simulink model "sk_R3GDL_2017"  (Simulink 9.1)
settings: Solver=ode45  StartTime=0.0  StopTime=20  MaxStep=1e-3  RelTol=1e-3  EnableMultiTasking=on
values from neighbouring files (symbols this model uses):
  A11 = 0.5    [Estimacion_Parametros_Ideal.m]    (also in Estimacion_Parametros_Real.m = 3; graficas.m)
  A12 = .5    (= 0.5)    [Estimacion_Parametros_Ideal.m]    (also in Estimacion_Parametros_Real.m = 3; graficas.m)
  F11 = 5    [Estimacion_Parametros_Ideal.m]    (also in Estimacion_Parametros_Real.m; graficas.m)
  F12 = 3    [Estimacion_Parametros_Ideal.m]    (also in Estimacion_Parametros_Real.m = 15; graficas.m)
  Ph11 = 0.5    [Estimacion_Parametros_Ideal.m]    (also in Estimacion_Parametros_Real.m = 0; graficas.m)
  Ph12 = 0    [Estimacion_Parametros_Ideal.m]    (also in Estimacion_Parametros_Real.m; graficas.m)
  Tm = 0.001    [Estimacion_Parametros_Ideal.m]    (also in Estimacion_Parametros_Real.m; graficas.m)
settings Model: Creator=mortega  LastModifiedBy=rafap  ExtModeTrigMode=oneshot  ExtModeArmWhenConnect=off
settings DataIOCC: SignalLoggingSaveFormat=ModelDataLogs
settings OptimizationCC: BlockReduction=off  BooleanDataType=off  ExpressionDepthLimit=2147483647  InitFltsAndDblsToZero=on
settings DebuggingCC: SaveWithParameterizedLinksMsg=none  SignalResolutionControl=TryResolveAllWithWarning  MultiTaskDSMMsg=warning  MultiTaskCondExecSysMsg=none  FcnCallInpInsideContextMsg=warning  StateNameClashWarn=warning
settings HardwareCC: TargetUnknown=on
settings GRTTargetCC: TargetFcnLib=ansi_tfl_tmw.mat

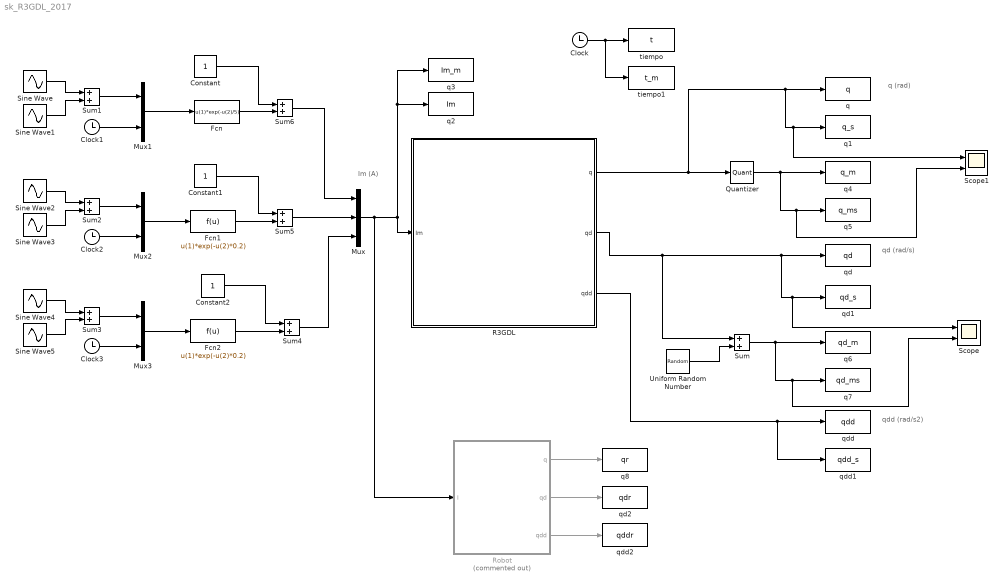
== system sk_R3GDL_2017 ==
  note: Im (A)
  note: q (rad)
  note: qd (rad/s)
  note: qdd (rad/s2)
  Clock{,1..3} (4 alike) : Clock
  Constant : Constant
  Constant1 : Constant
  Constant2 : Constant
  Fcn : Fcn  Expr=u(1)*exp(-u(2)/5)
  Fcn1 : Fcn  Expr=u(1)*exp(-u(2)*0.2)
  Fcn2 : Fcn  Expr=u(1)*exp(-u(2)*0.2)
  Mux : Mux  Inputs=3
  Mux1 : Mux  Inputs=2
  Mux2 : Mux  Inputs=2
  Mux3 : Mux  Inputs=2
  Quantizer : Quantizer  QuantizationInterval=(2*pi)/1024
  R3GDL : Subsystem  mask(Control y Programación de Robots (4 GIERM)){NGrupo=13, q1_ini=0, q2_ini=0, q3_ini=0, Bl_q1=off, Bl_q2=off, Bl_q3=off, AccionamientoDirecto=on}
      mask prompts: NGrupo "Nº de GRUPO"; q1_ini "q1 inicial  (rad)"; q2_ini "q2 inicial (rad)"; q3_ini "q3_inicial (rad)"; Bl_q1 "Bloqueo q1"; Bl_q2 "Bloqueo q2"; Bl_q3 "Bloqueo q3"; AccionamientoDirecto "Accionamiento directo"
      mask help: Robot de 3 grados de libertad RRR
      mask Display:
      | image(imread('R3GDL_RRR.JPG'));
      | port_label('output', 1, 'q');
      | port_label('output', 2, 'qd');
      | port_label('output', 3, 'qdd');
      | port_label('input', 1, 'Im')
  Robot : Subsystem  Commented=on
  Scope : Scope  NumInputPorts=2
  Scope1 : Scope  NumInputPorts=2
  Sine Wave : Sin  Amplitude=A11  Frequency=F11  Phase=Ph11  SampleTime=0
  Sine Wave1 : Sin  Amplitude=A12  Frequency=F12  Phase=Ph12  SampleTime=0
  Sine Wave2 : Sin  Amplitude=A11  Frequency=F11  Phase=Ph11  SampleTime=0
  Sine Wave3 : Sin  Amplitude=A12  Frequency=F12  Phase=Ph12  SampleTime=0
  Sine Wave4 : Sin  Amplitude=A11  Frequency=F11  Phase=Ph11  SampleTime=0
  Sine Wave5 : Sin  Amplitude=A12  Frequency=F12  Phase=Ph12  SampleTime=0
  Sum{,1..6} (7 alike) : Sum
  Uniform Random Number : UniformRandomNumber  Minimum=-0.005  Maximum=0.005  SampleTime=Tm
  q : ToWorkspace  VariableName=q  SampleTime=-1
  q1 : ToWorkspace  VariableName=q_s  SampleTime=Tm
  q2 : ToWorkspace  VariableName=Im  SampleTime=-1
  q3 : ToWorkspace  VariableName=Im_m  SampleTime=Tm
  q4 : ToWorkspace  VariableName=q_m  SampleTime=-1
  q5 : ToWorkspace  VariableName=q_ms  SampleTime=Tm
  q6 : ToWorkspace  VariableName=qd_m  SampleTime=-1
  q7 : ToWorkspace  VariableName=qd_ms  SampleTime=Tm
  q8 : ToWorkspace  VariableName=qr  SampleTime=-1
  qd : ToWorkspace  VariableName=qd  SampleTime=-1
  qd1 : ToWorkspace  VariableName=qd_s  SampleTime=Tm
  qd2 : ToWorkspace  VariableName=qdr  SampleTime=-1
  qdd : ToWorkspace  VariableName=qdd  SampleTime=-1
  qdd1 : ToWorkspace  VariableName=qdd_s  SampleTime=Tm
  qdd2 : ToWorkspace  VariableName=qddr  SampleTime=-1
  tiempo : ToWorkspace  VariableName=t  SampleTime=-1
  tiempo1 : ToWorkspace  VariableName=t_m  SampleTime=Tm
  wires:
  Clock/1 -> tiempo1/1, tiempo/1
  Mux/1 -> Robot/1(I), q3/1, q2/1, R3GDL/1(Im)
  R3GDL/2(qd) -> Sum/1, Scope/1, qd1/1, qd/1
  R3GDL/3(qdd) -> qdd1/1, qdd/1
  Uniform Random Number/1 -> Sum/2
  Sine Wave/1 -> Sum1/1
  Sine Wave1/1 -> Sum1/2
  Sine Wave2/1 -> Sum2/1
  Sine Wave3/1 -> Sum2/2
  Sine Wave4/1 -> Sum3/1
  Sine Wave5/1 -> Sum3/2
  Sum1/1 -> Mux1/1
  Clock1/1 -> Mux1/2
  Clock2/1 -> Mux2/2
  Sum2/1 -> Mux2/1
  Clock3/1 -> Mux3/2
  Sum3/1 -> Mux3/1
  Mux1/1 -> Fcn/1
  Mux2/1 -> Fcn1/1
  Mux3/1 -> Fcn2/1
  Fcn/1 -> Sum6/2
  Fcn1/1 -> Sum5/2
  Fcn2/1 -> Sum4/2
  Sum5/1 -> Mux/2
  Sum6/1 -> Mux/1
  Sum4/1 -> Mux/3
  Constant/1 -> Sum6/1
  Constant1/1 -> Sum5/1
  Constant2/1 -> Sum4/1
  Robot/3(qdd) -> qdd2/1
  Robot/1(q) -> q8/1
  Robot/2(qd) -> qd2/1
  Sum/1 -> Scope/2, q7/1, q6/1
  Quantizer/1 -> Scope1/2, q5/1, q4/1
  R3GDL/1(q) -> Scope1/1, q1/1, q/1, Quantizer/1

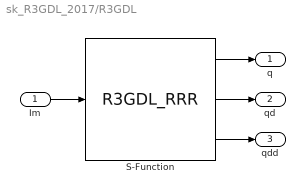
== system sk_R3GDL_2017/R3GDL ==
  Im : Inport
  S-Function : S-Function  FunctionName=R3GDL_RRR  Parameters=[q1_ini; q2_ini; q3_ini]; [Bl_q1; Bl_q2; Bl_q3]; AccionamientoDirecto; NGrupo  SFunctionDeploymentMode=off  EnableBusSupport=off
  q : Outport
  qd : Outport  Port=2
  qdd : Outport  Port=3
  wires:
  Im/1 -> S-Function/1
  S-Function/1 -> q/1
  S-Function/2 -> qd/1
  S-Function/3 -> qdd/1

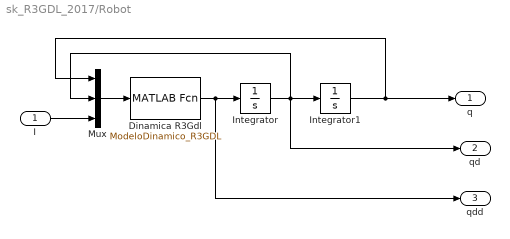
== system sk_R3GDL_2017/Robot ==
  I : Inport
  Dinamica R3Gdl : MATLABFcn  MATLABFcn=ModeloDinamico_R3GDL
  Integrator : Integrator  InitialCondition=[0;0;0]
  Integrator1 : Integrator  InitialCondition=[0;0;0]
  Mux : Mux  Inputs=3
  q : Outport
  qd : Outport  Port=2
  qdd : Outport  Port=3
  wires:
  Mux/1 -> Dinamica R3Gdl/1
  Dinamica R3Gdl/1 -> Integrator/1, qdd/1
  Integrator/1 -> Integrator1/1, qd/1, Mux/2
  Integrator1/1 -> q/1, Mux/1
  I/1 -> Mux/3
